simulink model "buildex"  (R2017a)
settings: Solver=ode45  StartTime=0.0  StopTime=10.0  RelTol=1e-3
settings Model: Creator=sansh  LastModifiedBy=sansh

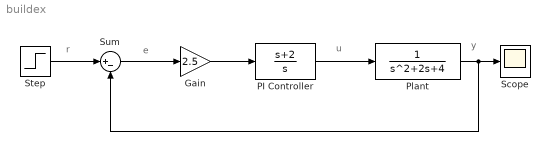
== system buildex ==
  note: y
  note: u
  note: e
  note: r
  Gain : Gain  Gain=2.5
  PI Controller : TransferFcn  Numerator=[1 2]  Denominator=[1 0]
  Plant : TransferFcn  Denominator=[1 2 4]
  Scope : Scope
  Step : Step  SampleTime=0
  Sum : Sum  Inputs=|+-
  wires:
  Step/1 -> Sum/1
  Sum/1 -> Gain/1
  Gain/1 -> PI Controller/1
  Plant/1 -> Sum/2, Scope/1
  PI Controller/1 -> Plant/1
